simulink model "SPWM_jisuan"  (R2024b)
settings: Solver=VariableStepAuto  StartTime=1  StopTime=2  RelTol=1e-3
undefined symbols (not defined in the file): Down, Up
libraries: spsControlledVoltageSourceLib x3, eePwmGenerator x3, spsPermanentMagnetSynchronousMachineLib x1, sps_lib x1
settings Model: Creator=刘炳宏  LastModifiedBy=刘炳宏

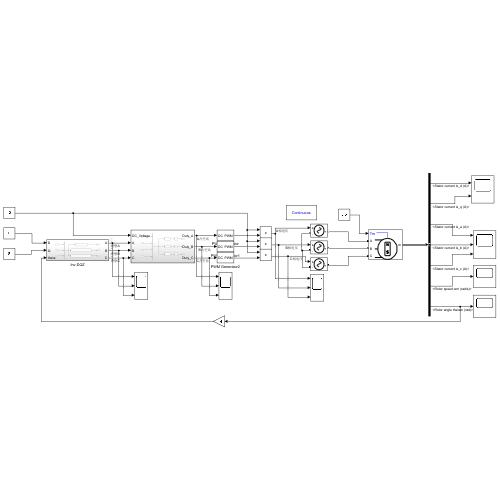
[thumbnail: Simulink's stored preview of the top-level diagram]
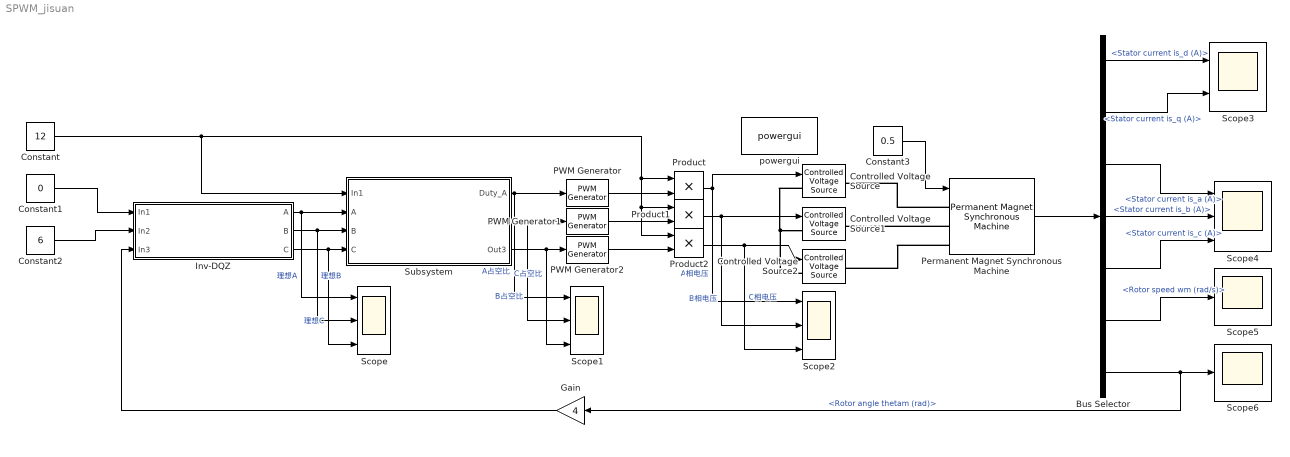
== system SPWM_jisuan ==
  Bus Selector : BusSelector  OutputSignals=Stator current is_d (A),Stator current is_q (A),Stator current is_a (A),Stator current is_b (A),Stator current is_c (A),Rotor speed wm (rad/s),Rotor angle thetam (rad)
  Constant : Constant  Value=12
  Constant1 : Constant  Value=0
  Constant2 : Constant  Value=6
  Constant3 : Constant  Value=0.5
  Controlled Voltage Source : spsControlledVoltageSourceLib/Controlled Voltage Source  Initialize=on  Source_Type=DC  Amplitude=0  Phase=0  Frequency=0  Measurements=None
  Controlled Voltage Source1 : spsControlledVoltageSourceLib/Controlled Voltage Source  Initialize=on  Source_Type=DC  Amplitude=0  Phase=0  Frequency=0  Measurements=None
  Controlled Voltage Source2 : spsControlledVoltageSourceLib/Controlled Voltage Source  Initialize=on  Source_Type=DC  Amplitude=0  Phase=0  Frequency=0  Measurements=None
  Gain : Gain  Gain=4
  Inv-DQZ : Subsystem
  PWM Generator : eePwmGenerator/PWM Generator  CarrCount=Up-Down  Tper=0.0001  Tdelay=0  Ts=5e-6
  PWM Generator1 : eePwmGenerator/PWM Generator  CarrCount=Up-Down  Tper=0.0001  Tdelay=0  Ts=5e-6
  PWM Generator2 : eePwmGenerator/PWM Generator  CarrCount=Up-Down  Tper=0.0001  Tdelay=0  Ts=5e-6
  Permanent Magnet Synchronous Machine : spsPermanentMagnetSynchronousMachineLib/Permanent Magnet Synchronous Machine  NbPhases=3  FluxDistribution=Sinusoidal  RotorType=Round  MechanicalLoad=Torque Tm  PresetModel=No  ShowDetailedParameters=on  MeasurementBus=off  Resistance=0.18  Inductance=8.5e-3  dqInductances=[8.5e-3,8.5e-3]  La=8.5e-3  MachineConstant=Flux linkage established by magnets (V.s)  Flux=0.074147  VoltageCst=53.7951  TorqueCst=0.44488  Flat=120  Mechanical=[0.00062 0.0003505 4 0]  PolePairs=4  InitialConditions=[0,1, 0,0]  InitialConditions5ph=[0 0 0 0 0 0]  RefAngle=Aligned with phase A axis (original Park)  IterativeDiscreteModel=Trapezoidal non iterative  TsBlock=-1  TsPowergui=0
  Product : Product
  Product1 : Product
  Product2 : Product
  Scope{,1..2,4} (4 alike) : Scope  NumInputPorts=3
  Scope3 : Scope  NumInputPorts=2
  Scope5 : Scope
  Scope6 : Scope
  Subsystem : Subsystem
  powergui : sps_lib/powergui  Priority=1  SimulationMode=Continuous  SampleTime=50e-6  frequency=60  Iterations=50  frequencyindice=0  Pbase=100e6  ErrMax=1e-4  UnitsV=kV  UnitsW=MW  buscounter=0  FunctionMessages=off  echomessages=off  EnableUseOfTLC=off  CurrentSourceSwitches=off  DisableSnubberDevices=off  DisableRonSwitches=off  DisableVfSwitches=off  DisplayEquations=off  AutomaticDiscreteSolvers=off  SolverType=Tustin/Backward Euler (TBE)  Interpol=off  ExternalGateDelay=off  methode=off  Ts=100  x0status=blocks  SPID=on  SwTol=0  HookPort=off  NonlinearTolerance=1e-4  nMaxIteration=100  ContinueOnMaxIteration=off  RestoreLinks=warning  ResistiveCurrentMeasurement=off  Frange=[0:2:500]  Ylog=off  Xlog=on  ShowGrid=off  save=off  variable=ZData  structure=0  ZoomFFT=off  StartTime=0.0  cycles=1  DisplayStyle=1  fundamental=60  FreqAxis=off  MaxFrequency=1000  frequencyindicesteady=1  RmsSteady=1  display=off
  wires:
  Inv-DQZ/2(B) -> Scope/2, Subsystem/3(B)  "理想B"
  Inv-DQZ/3(C) -> Scope/3, Subsystem/4(C)  "理想C"
  Inv-DQZ/1(A) -> Scope/1, Subsystem/2(A)  "理想A"
  Subsystem/1(Duty_A) -> PWM Generator/1, Scope1/1  "A占空比"
  Subsystem/2(Out2) -> PWM Generator1/1, Scope1/2  "B占空比"
  Subsystem/3(Out3) -> PWM Generator2/1, Scope1/3  "C占空比"
  PWM Generator/1 -> Product/2
  PWM Generator1/1 -> Product1/2
  PWM Generator2/1 -> Product2/2
  Constant/1 -> Product2/1, Product1/1, Product/1, Subsystem/1(In1)
  Constant1/1 -> Inv-DQZ/1(In1)
  Constant2/1 -> Inv-DQZ/2(In2)
  Constant3/1 -> Permanent Magnet Synchronous Machine/1
  Product/1 -> Scope2/1, Controlled Voltage Source/1  "A相电压"
  Product1/1 -> Scope2/2, Controlled Voltage Source1/1  "B相电压"
  Product2/1 -> Scope2/3, Controlled Voltage Source2/1  "C相电压"
  Permanent Magnet Synchronous Machine/1 -> Bus Selector/1
  Bus Selector/1 -> Scope3/1  "<Stator current is_d (A)>"
  Bus Selector/2 -> Scope3/2  "<Stator current is_q (A)>"
  Bus Selector/4 -> Scope4/2  "<Stator current is_b (A)>"
  Bus Selector/3 -> Scope4/1  "<Stator current is_a (A)>"
  Bus Selector/5 -> Scope4/3  "<Stator current is_c (A)>"
  Bus Selector/6 -> Scope5/1  "<Rotor speed wm (rad/s)>"
  Bus Selector/7 -> Gain/1, Scope6/1  "<Rotor angle thetam (rad)>"
  Gain/1 -> Inv-DQZ/3(In3)
  connections:
  Permanent Magnet Synchronous Machine/LConn2 -- Controlled Voltage Source1/RConn1
  Permanent Magnet Synchronous Machine/LConn3 -- Controlled Voltage Source2/RConn1
  Permanent Magnet Synchronous Machine/LConn1 -- Controlled Voltage Source/RConn1
  Controlled Voltage Source/LConn1 -- Controlled Voltage Source2/LConn1 -- Controlled Voltage Source1/LConn1

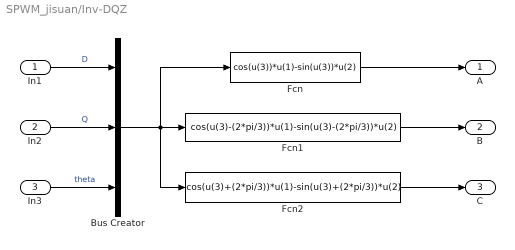
== system SPWM_jisuan/Inv-DQZ ==
  In1 : Inport
  In2 : Inport  Port=2
  In3 : Inport  Port=3
  Bus Creator : BusCreator  Inputs=3
  Fcn : Fcn  Expr=cos(u(3))*u(1)-sin(u(3))*u(2)
  Fcn1 : Fcn  Expr=cos(u(3)-(2*pi/3))*u(1)-sin(u(3)-(2*pi/3))*u(2)
  Fcn2 : Fcn  Expr=cos(u(3)+(2*pi/3))*u(1)-sin(u(3)+(2*pi/3))*u(2)
  A : Outport
  B : Outport  Port=2
  C : Outport  Port=3
  wires:
  In3/1 -> Bus Creator/3  "theta"
  In2/1 -> Bus Creator/2  "Q"
  In1/1 -> Bus Creator/1  "D"
  Bus Creator/1 -> Fcn/1, Fcn1/1, Fcn2/1
  Fcn/1 -> A/1
  Fcn1/1 -> B/1
  Fcn2/1 -> C/1

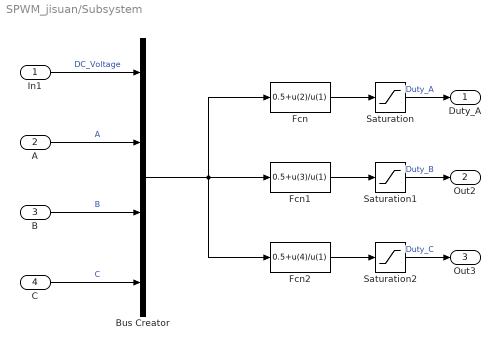
== system SPWM_jisuan/Subsystem ==
  In1 : Inport
  A : Inport  Port=2
  B : Inport  Port=3
  C : Inport  Port=4
  Bus Creator : BusCreator  Inputs=4
  Fcn : Fcn  Expr=0.5+u(2)/u(1)
  Fcn1 : Fcn  Expr=0.5+u(3)/u(1)
  Fcn2 : Fcn  Expr=0.5+u(4)/u(1)
  Saturation : Saturate  UpperLimit=1  LowerLimit=0
  Saturation1 : Saturate  UpperLimit=1  LowerLimit=0
  Saturation2 : Saturate  UpperLimit=1  LowerLimit=0
  Duty_A : Outport
  Out2 : Outport  Port=2
  Out3 : Outport  Port=3
  wires:
  In1/1 -> Bus Creator/1  "DC_Voltage"
  A/1 -> Bus Creator/2  "A"
  B/1 -> Bus Creator/3  "B"
  C/1 -> Bus Creator/4  "C"
  Fcn/1 -> Saturation/1
  Bus Creator/1 -> Fcn/1, Fcn2/1, Fcn1/1
  Saturation/1 -> Duty_A/1  "Duty_A"
  Saturation1/1 -> Out2/1  "Duty_B"
  Fcn1/1 -> Saturation1/1
  Saturation2/1 -> Out3/1  "Duty_C"
  Fcn2/1 -> Saturation2/1
